simulink library "FVTMCU_lib"  (R2024a)
settings: Solver=VariableStepAuto  StartTime=0.0  StopTime=10.0  RelTol=1e-3
undefined symbols (not defined in the file): FALSE, MINUSONE_FLOAT, ONE_FLOAT, TRUE, ZERO_FLOAT
libraries: simulink x1
settings Model: Creator=FVT22063  LastModifiedBy=FVT22063

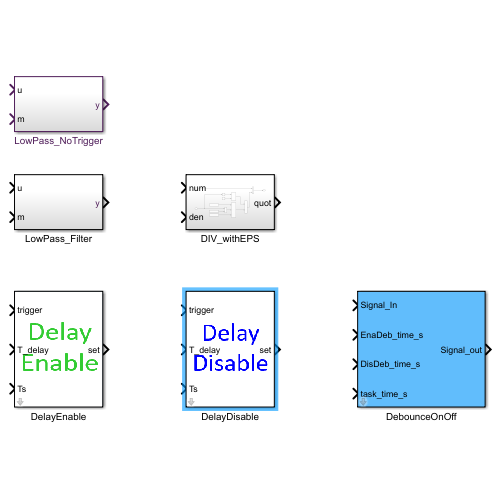
[thumbnail: Simulink's stored preview of the top-level diagram]
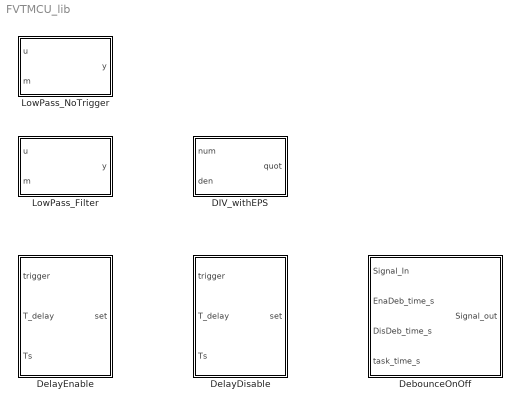
== system FVTMCU_lib ==
  DIV_withEPS : Subsystem
  DebounceOnOff : Subsystem  mask(Debounced Enable and Disable){}
      mask help:
      | Enable with debounce time
      | Disable with debounce time
  DelayDisable : Subsystem  mask(DelayDisable){}
      mask help: Delay Disable function
      mask Display: image('DelayDisable.png');
  DelayEnable : Subsystem  mask(DelayEnable){}
      mask help: Delay enable funcion.
      mask Display: image('DelayEnable.png');
  LowPass_Filter : Subsystem
  LowPass_NoTrigger : Subsystem

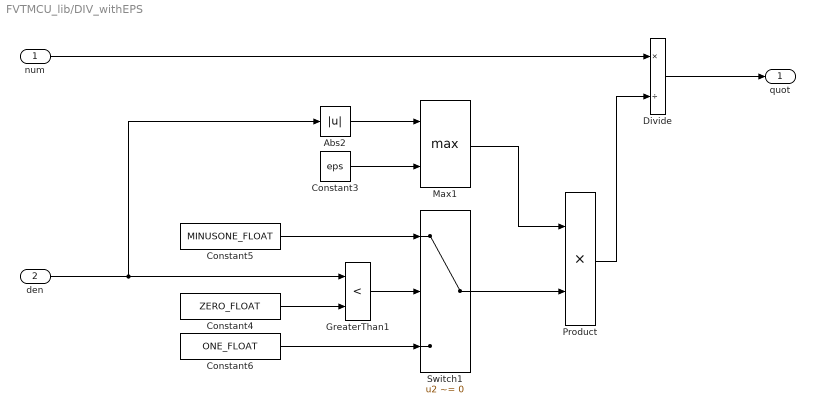
== system FVTMCU_lib/DIV_withEPS ==
  num : Inport
  den : Inport  Port=2
  Abs2 : Abs  SaturateOnIntegerOverflow=off
  Constant3 : Constant  Value=eps
  Constant4 : Constant  Value=ZERO_FLOAT  OutDataTypeStr=int8  SampleTime=-1
  Constant5 : Constant  Value=MINUSONE_FLOAT  OutDataTypeStr=int8  SampleTime=-1
  Constant6 : Constant  Value=ONE_FLOAT  OutDataTypeStr=int8  SampleTime=-1
  Divide : Product  Inputs=*/  OutDataTypeStr=int8  RndMeth=Zero
  GreaterThan1 : RelationalOperator  Operator=<  OutDataTypeStr=boolean  RndMeth=Simplest  InputSameDT=off
  Max1 : MinMax  Function=max  Inputs=2
  Product : Product
  Switch1 : Switch  Criteria=u2 ~= 0  SaturateOnIntegerOverflow=off  InputSameDT=off
  quot : Outport
  wires:
  Divide/1 -> quot/1
  Product/1 -> Divide/2
  num/1 -> Divide/1
  Constant3/1 -> Max1/2
  Abs2/1 -> Max1/1
  Constant4/1 -> GreaterThan1/2
  den/1 -> Abs2/1, GreaterThan1/1
  GreaterThan1/1 -> Switch1/2
  Constant5/1 -> Switch1/1
  Max1/1 -> Product/1
  Switch1/1 -> Product/2
  Constant6/1 -> Switch1/3

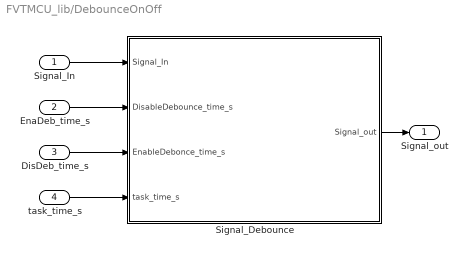
== system FVTMCU_lib/DebounceOnOff ==
  Signal_In : Inport
  EnaDeb_time_s : Inport  Port=2
  DisDeb_time_s : Inport  Port=3
  task_time_s : Inport  Port=4
  Signal_Debounce : Stateflow chart  TreatAsAtomicUnit=on
  Signal_out : Outport
  wires:
  EnaDeb_time_s/1 -> Signal_Debounce/2(DisableDebounce_time_s)
  Signal_In/1 -> Signal_Debounce/1(Signal_In)
  Signal_Debounce/1(Signal_out) -> Signal_out/1
  task_time_s/1 -> Signal_Debounce/4(task_time_s)
  DisDeb_time_s/1 -> Signal_Debounce/3(EnableDebonce_time_s)

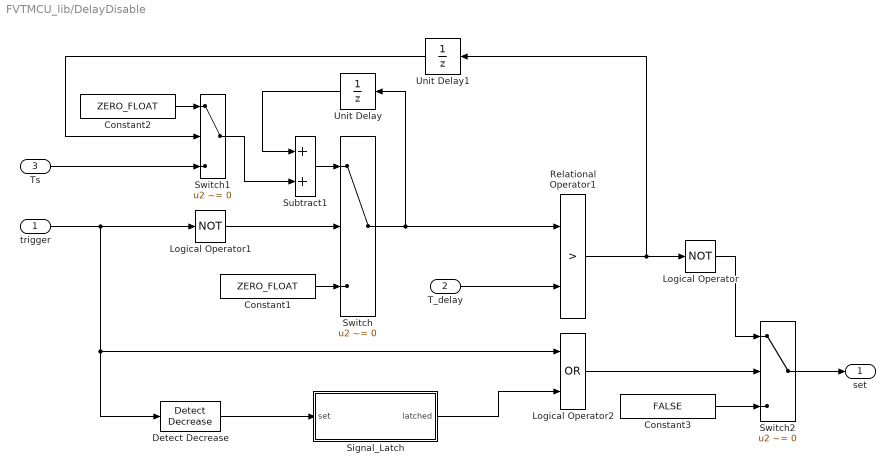
== system FVTMCU_lib/DelayDisable ==
  trigger : Inport
  T_delay : Inport  Port=2
  Ts : Inport  Port=3
  Constant1 : Constant  Value=ZERO_FLOAT
  Constant2 : Constant  Value=ZERO_FLOAT
  Constant3 : Constant  Value=FALSE
  Detect Decrease : simulink/Logic and Bit Operations/Detect Decrease  vinit=0.0  OutDataTypeStr=boolean
  Logical Operator : Logic  Operator=NOT  AllPortsSameDT=off  OutDataTypeStr=boolean
  Logical Operator1 : Logic  Operator=NOT  AllPortsSameDT=off  OutDataTypeStr=boolean
  Logical Operator2 : Logic  Operator=OR  AllPortsSameDT=off  OutDataTypeStr=boolean
  Relational Operator1 : RelationalOperator  Operator=>  OutDataTypeStr=boolean  InputSameDT=off
  Signal_Latch : Subsystem
  Subtract1 : Sum
  Switch : Switch  Criteria=u2 ~= 0  SaturateOnIntegerOverflow=off  InputSameDT=off
      settings: AttributesFormatString=<%<Criteria>>
  Switch1 : Switch  Criteria=u2 ~= 0  SaturateOnIntegerOverflow=off  InputSameDT=off
      settings: AttributesFormatString=<%<Criteria>>
  Switch2 : Switch  Criteria=u2 ~= 0  SaturateOnIntegerOverflow=off  InputSameDT=off
  Unit Delay : UnitDelay  SampleTime=-1  HasFrameUpgradeWarning=on
      settings: AttributesFormatString=<intial = %<X0>>
  Unit Delay1 : UnitDelay  InitialCondition=FALSE  SampleTime=-1  HasFrameUpgradeWarning=on
      settings: AttributesFormatString=<intial = %<X0>>
  set : Outport
  wires:
  Unit Delay1/1 -> Switch1/2
  Constant2/1 -> Switch1/1
  Ts/1 -> Switch1/3
  Switch1/1 -> Subtract1/2
  Unit Delay/1 -> Subtract1/1
  T_delay/1 -> Relational Operator1/2
  Constant1/1 -> Switch/3
  Switch/1 -> Unit Delay/1, Relational Operator1/1
  Subtract1/1 -> Switch/1
  Relational Operator1/1 -> Unit Delay1/1, Logical Operator/1
  Logical Operator1/1 -> Switch/2
  trigger/1 -> Detect Decrease/1, Logical Operator2/1, Logical Operator1/1
  Detect Decrease/1 -> Signal_Latch/1(set)
  Signal_Latch/1(latched) -> Logical Operator2/2
  Constant3/1 -> Switch2/3
  Switch2/1 -> set/1
  Logical Operator/1 -> Switch2/1
  Logical Operator2/1 -> Switch2/2

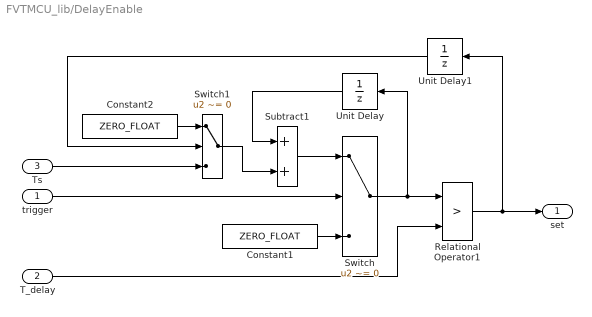
== system FVTMCU_lib/DelayEnable ==
  trigger : Inport
  T_delay : Inport  Port=2
  Ts : Inport  Port=3
  Constant1 : Constant  Value=ZERO_FLOAT
  Constant2 : Constant  Value=ZERO_FLOAT
  Relational Operator1 : RelationalOperator  Operator=>  OutDataTypeStr=boolean  InputSameDT=off
  Subtract1 : Sum
  Switch : Switch  Criteria=u2 ~= 0  SaturateOnIntegerOverflow=off  InputSameDT=off
      settings: AttributesFormatString=<%<Criteria>>
  Switch1 : Switch  Criteria=u2 ~= 0  SaturateOnIntegerOverflow=off  InputSameDT=off
      settings: AttributesFormatString=<%<Criteria>>
  Unit Delay : UnitDelay  SampleTime=-1  HasFrameUpgradeWarning=on
      settings: AttributesFormatString=<intial = %<X0>>
  Unit Delay1 : UnitDelay  InitialCondition=FALSE  SampleTime=-1  HasFrameUpgradeWarning=on
      settings: AttributesFormatString=<intial = %<X0>>
  set : Outport
  wires:
  Unit Delay1/1 -> Switch1/2
  Constant2/1 -> Switch1/1
  Ts/1 -> Switch1/3
  Switch1/1 -> Subtract1/2
  Unit Delay/1 -> Subtract1/1
  Relational Operator1/1 -> Unit Delay1/1, set/1
  trigger/1 -> Switch/2
  T_delay/1 -> Relational Operator1/2
  Constant1/1 -> Switch/3
  Switch/1 -> Unit Delay/1, Relational Operator1/1
  Subtract1/1 -> Switch/1

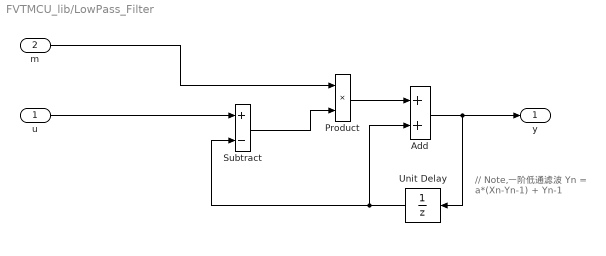
== system FVTMCU_lib/LowPass_Filter ==
  note: // Note,一阶低通滤波
      | Yn = a*(Xn-Yn-1) + Yn-1
  u : Inport
      settings: AttributesFormatString=%<OutDataTypeStr>
  m : Inport  Port=2
      settings: AttributesFormatString=%<OutDataTypeStr>
  Add : Sum
  Product : Product
  Subtract : Sum  Inputs=+-
  Unit Delay : UnitDelay  SampleTime=-1  HasFrameUpgradeWarning=on
  y : Outport  VectorParamsAs1DForOutWhenUnconnected=off
      settings: AttributesFormatString=%<OutDataTypeStr>
  wires:
  Subtract/1 -> Product/2
  m/1 -> Product/1
  u/1 -> Subtract/1
  Unit Delay/1 -> Add/2, Subtract/2
  Product/1 -> Add/1
  Add/1 -> Unit Delay/1, y/1

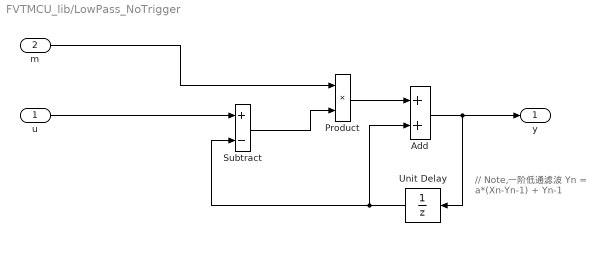
== system FVTMCU_lib/LowPass_NoTrigger ==
  note: // Note,一阶低通滤波
      | Yn = a*(Xn-Yn-1) + Yn-1
  u : Inport
      settings: AttributesFormatString=%<OutDataTypeStr>
  m : Inport  Port=2
      settings: AttributesFormatString=%<OutDataTypeStr>
  Add : Sum
  Product : Product
  Subtract : Sum  Inputs=+-
  Unit Delay : UnitDelay  SampleTime=-1  HasFrameUpgradeWarning=on
  y : Outport  VectorParamsAs1DForOutWhenUnconnected=off
      settings: AttributesFormatString=%<OutDataTypeStr>
  wires:
  Product/1 -> Add/1
  m/1 -> Product/1
  Unit Delay/1 -> Add/2, Subtract/2
  Subtract/1 -> Product/2
  Add/1 -> Unit Delay/1, y/1
  u/1 -> Subtract/1

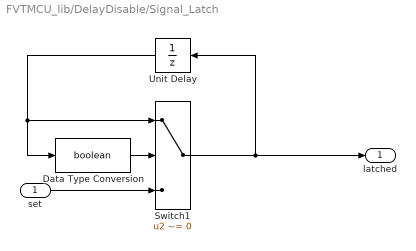
== system FVTMCU_lib/DelayDisable/Signal_Latch ==
  set : Inport
  Data Type Conversion : DataTypeConversion  OutDataTypeStr=boolean  SaturateOnIntegerOverflow=off  RndMeth=Floor
  Switch1 : Switch  Criteria=u2 ~= 0  Threshold=0.5  SaturateOnIntegerOverflow=off  InputSameDT=off
      settings: AttributesFormatString=<Criteria=%<Criteria>>
  Unit Delay : UnitDelay  SampleTime=-1  HasFrameUpgradeWarning=on
  latched : Outport
  wires:
  Switch1/1 -> latched/1, Unit Delay/1
  Unit Delay/1 -> Data Type Conversion/1, Switch1/1
  Data Type Conversion/1 -> Switch1/2
  set/1 -> Switch1/3

== stateflow chart FVTMCU_lib/DebounceOnOff/Signal_Debounce ==
  (default) -> (junction 25)
  (junction 25) -> (junction 20)
  (junction 20) -> (junction 29) [order 2] : [Signal_In==FALSE]
  (junction 20) -> (junction 27) [order 1] : [Signal_In==TRUE]
  (junction 29) -> (junction 30) : {count2 += task_time_s;
      |  count1 = 0;}
  (junction 20) -> (junction 24) [order 3]
  (junction 27) -> (junction 28) : {count1 += task_time_s;
      |  count2 = 0;}
  (junction 30) -> (junction 24)
  (junction 28) -> (junction 24)
  (junction 24) -> (junction 21)
  (junction 21) -> (junction 31) [order 2] : [count2 >= DisableDebounce_time_s]
  (junction 21) -> (junction 33) [order 1] : [count1 >= EnableDebonce_time_s]
  (junction 31) -> (junction 32) : {count2 = DisableDebounce_time_s;
      | Signal_out=FALSE;}
  (junction 21) -> (junction 22) [order 3]
  (junction 33) -> (junction 34) : {count1 = EnableDebonce_time_s;
      | Signal_out = TRUE;}
  (junction 32) -> (junction 22)
  (junction 34) -> (junction 22)
  (junction 22) -> (junction 26)
  (junction 26) -> (junction 23)
  data: Signal_In input boolean; Signal_out output boolean =0; TRUE parameter boolean; FALSE parameter boolean; DisableDebounce_time_s input single; EnableDebonce_time_s input single; task_time_s input; count1 local single; count2 local single
